simulink model "mppt1"  (R2026a)
settings: Solver=VariableStepAuto
libraries: fl_lib x9, nesl_utility x5, ee_lib x3, batt_lib x2, batteryecm_lib x1, eePwmGenerator x1
(part 1 of 2)
settings Model: Creator=Patrick  LastModifiedBy=caden

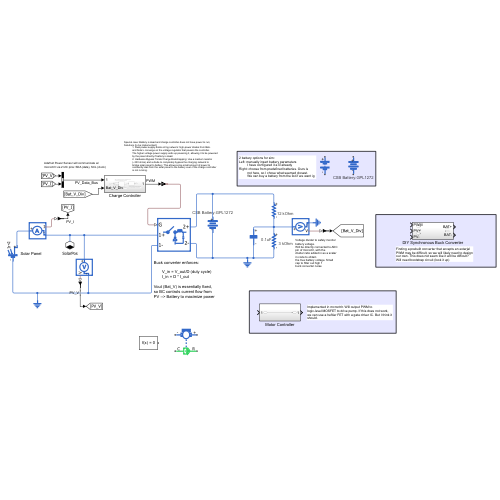
[thumbnail: Simulink's stored preview of the top-level diagram]
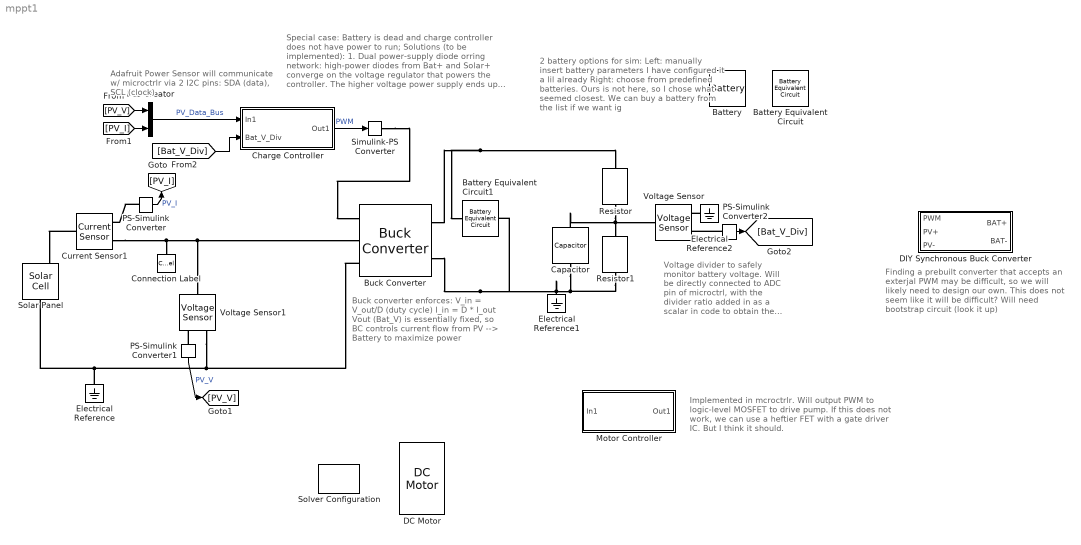
== system mppt1 ==
  note: Special case: Battery is dead and charge controller does not have power to run;
      | Solutions (to be implemented):
      | 1. Dual power-supply diode orring network: high-power diodes from Bat+
      | and Solar+ converge on the voltage regulator that powers the controller.
      | The higher voltage power supply ends up powering it, allowing it to be powered
      | by the panel directly if battery is dead.
      | 2. Hardware Bypass Trickle Charge Bootstrapping: Use a medium resistor
      | (~330 ohms) and a diode to completely bypass the charging network to
      | bridge solar panel to battery. This allows some small amount of power to
      | constantly leak from the solar panel to the battery even if the charge controller
      | is not running.
  note: Implemented in mcroctrlr. Will output PWM to
      | logic-level MOSFET to drive pump. If this does not work,
      | we can use a heftier FET with a gate driver IC. But I think it
      | should.
  note: Finding a prebuilt converter that accepts an exterjal
      | PWM may be difficult, so we will likely need to design
      | our own. This does not seem like it will be difficult?
      | Will need bootstrap circuit (look it up)
  note: Voltage divider to safely monitor battery voltage.
      | Will be directly connected to ADC pin of microctrl, with the
      | divider ratio added in as a scalar in code to obtain
      | the true battery voltage. Small cap to filter out high f
      | buck converter noise
  note: 2 battery options for sim:
      | Left: manually insert battery parameters
      | I have configured it a lil already
      | Right: choose from predefined batteries. Ours is
      | not here, so I chose what seemed closest.
      | We can buy a battery from the list if we want ig
  note: Adafruit Power Sensor will communicate w/
      | microctrlr via 2 I2C pins: SDA (data), SCL (clock)
  note: Buck converter enforces:
      |
      | 	V_in = V_out/D (duty cycle)
      | 	I_in = D * I_out
      |
      | Vout (Bat_V) is essentially fixed,
      | so BC controls current flow from
      | PV --> Battery to maximize power
  Battery : batteryecm_lib/Battery  Vnom=12 V  prm_dir=simscape.enum.battery.prm_dir.disabled  R1_dis=2 Ohm  R1_ch=2 Ohm  R1=25 mOhm  prm_AH=simscape.enum.battery.prm_AH.finite  AH=8 A*hr  V1=11 V  AH1=1.6 A*hr  prm_R2=simscape.enum.battery.prm_R2.disabled  R2=2000 Ohm  Tmeas=298.15 K  charge_measurement_port=simscape.enum.battery.enable.no  prm_dyn=simscape.enum.battery.prm_dyn.rc1  Rp1=0.005 Ohm  tau1=10 s  Rp2=0.005 Ohm  tau2=30 s  Rp3=0.005 Ohm  tau3=30 s  Rp4=0.005 Ohm  tau4=30 s  Rp5=0.005 Ohm  tau5=30 s  prm_fade=simscape.enum.battery.prm_fade.disabled  N_fade=100  AH_fade=45 A*hr  R1_fade=2.02 Ohm  R1_ch_fade=2.02 Ohm  V1_fade=10.35 V  prm_age=simscape.enum.battery.prm_age.disabled  prm_age_OCV=simscape.enum.battery.prm_age_OCV.OCV  OCV_age=0.9  SOC_age=60  Tmeas_age=298.15 K  delta_time_age_vec=[0] d  temperature_age_vec=[273] K  OCV_scaling_age=2.2134e6  OCV_offset_age=1.632e6  temp_exp_age=0.515833569 V  t_exp_age=0.75  Vnom_T2=12 V  R1_T2=2.2 Ohm  R1_T2_dis=2.2 Ohm  R1_T2_ch=2.2 Ohm  V1_T2=11.4 V  R2_T2=2200 Ohm  Rp1_T2=0.005 Ohm  tau1_T2=30 s  Rp2_T2=0.005 Ohm  tau2_T2=30 s  Rp3_T2=0.005 Ohm  tau3_T2=30 s  Rp4_T2=0.005 Ohm  tau4_T2=30 s  Rp5_T2=0.005 Ohm  tau5_T2=30 s  Tmeas2=273.15 K  thermal_port=simscape.enum.thermaleffects.omit  thermal_mass=30000 J/K  i_specify=off  i_priority=None  i=0 A  i_nominal_specify=off  i_nominal_value=1  i_nominal_unit=A  v_specify=off  v_priority=None  v=0 V  v_nominal_specify=off  v_nominal_value=1  v_nominal_unit=V  charge_specify=off  charge_priority=High  charge=50 A*hr  charge_nominal_specify=off  charge_nominal_value=1  charge_nominal_unit=A*hr  num_cycles_specify=off  num_cycles_priority=High  num_cycles=0  num_cycles_nominal_specify=off  num_cycles_nominal_value=1  num_cycles_nominal_unit=1  temperature_specify=off  temperature_priority=High  temperature=298.15 K  temperature_nominal_specify=off  temperature_nominal_value=1  temperature_nominal_unit=K
  Battery Equivalent Circuit : batt_lib/Cells/Battery Equivalent Circuit  PartSpecification="{\"CollectionId\":\"MW.SimscapeBattery\",\"CollectionVersion\":\"1.0.0\",\"DatasetId\":\"CSB Battery|GPL1272|simscape.battery.batteryEquivalentCircuit\",\"DisplayName\":\"CSB Battery:GPL1272\"}"  BatteryCapacity=7.2 % Datasheet derived hr*A  ThermalModel=simscape.battery.enum.cells.BatteryThermalModel.ConstantTemperature  ExtrapolationMethod=simscape.enum.extrapolation.linear  SOCBreakpoints=[0 0.02 0.04 0.06 0.08 0.1 0.12 0.14 0.16 0.18 0.2 0.22 0.24 0.26 0.28 0.3 0.32 0.34 0.36 0.38 0.4 0.42 0.44 0.46 0.48 0.5 0.52 0.54 0.56 0.58 0.6 0.62 0.64 0.66 0.68 0.7 0.72 0.74 0.76 0.78 0.8 0.82 0.84 0.86 0.88 0.9 0.92 0.94 0.96 0.98 1] % Datasheet derived  TemperatureBreakpoints=[25;30] % Parameter assumed degC  OpenCircuitVoltage=[10.55448 10.75925 10.91906 11.06757 11.18985 11.28642 11.36577 11.43656 11.50322 11.56016 11.61342 11.66505 11.71348 11.75917 11.80784 11.85717 11.90449 11.94971 11.9929 12.03397 12.07275 12.10969 12.14517 12.17949 12.21291 12.24568 12.27779 12.30916 12.3396 12.36887 12.39694 12.42373 12.4492 12.47369 12.49775 12.5218 12.54639 12.57213 12.59914 12.62744 12.65704 12.68789 12.71992 12.75327 12.78809 12.82459 12.86341 12.90404 12.94821 12.99301 13.04366] % Datasheet derived V  OpenCircuitVoltageThermal=[10.55448 10.55448;10.75925 10.75925;10.91906 10.91906;11.06757 11.06757;11.18985 11.18985;11.28642 11.28642;11.36577 11.36577;11.43656 11.43656;11.50322 11.50322;11.56016 11.56016;11.61342 11.61342;11.66505 11.66505;11.71348 11.71348;11.75917 11.75917;11.80784 11.80784;11.85717 11.85717;11.90449 11.90449;11.94971 11.94971;11.9929 11.9929;12.03397 12.03397;12.07275 12.07275;12.10969 12.10969;12.14517 12.14517;12.17949 12.17949;12.21291 12.21291;12.24568 12.24568;12.27779 12.27779;12.30916 12.30916;12.3396 12.3396;12.36887 12.36887;12.39694 12.39694;12.42373 12.42373;12.4492 12.4492;12.47369 12.47369;12.49775 12.49775;12.5218 12.5218;12.54639 12.54639;12.57213 12.57213;12.59914 12.59914;12.62744 12.62744;12.65704 12.65704;12.68789 12.68789;12.71992 12.71992;12.75327 12.75327;12.78809 12.78809;12.82459 12.82459;12.86341 12.86341;12.90404 12.90404;12.94821 12.94821;12.99301 12.99301;13.04366 13.04366] % Parameter assumed V  VoltageRange=[9.45 Inf] % Datasheet derived V  HysteresisModel=simscape.battery.enum.cells.HysteresisModel.none  MaximumHysteresisVoltage=[0, 0, 0, 0, 0, 0, 0] % Parameter not set V  InstantaneousHysteresisVoltage=[0, 0, 0, 0, 0, 0, 0] % Parameter not set V  HysteresisRate=0.1 % Parameter not set  MaximumHysteresisVoltageThermal=[0, 0, 0; 0, 0, 0; 0, 0, 0; 0, 0, 0; 0, 0, 0; 0, 0, 0; 0, 0, 0] % Parameter not set V  InstantaneousHysteresisVoltageThermal=[0, 0, 0; 0, 0, 0; 0, 0, 0; 0, 0, 0; 0, 0, 0; 0, 0, 0; 0, 0, 0] % Parameter not set V  HysteresisRateThermal=0.1 % Parameter not set  ResistanceSOCBreakpoints=[0 0.02 0.04 0.06 0.08 0.1 0.12 0.14 0.16 0.18 0.2 0.22 0.24 0.26 0.28 0.3 0.32 0.34 0.36 0.38 0.4 0.42 0.44 0.46 0.48 0.5 0.52 0.54 0.56 0.58 0.6 0.62 0.64 0.66 0.68 0.7 0.72 0.74 0.76 0.78 0.8 0.82 0.84 0.86 0.88 0.9 0.92 0.94 0.96 0.98 1] % Datasheet derived  ResistanceTemperatureBreakpoints=[25;30] % Parameter assumed degC  ResistanceCurrentBreakpoints=[-1, 0, 1] % Parameter not set A  CurrentDependence=simscape.battery.enum.cells.CurrentDependence.Disabled  R0=[0.4783 0.48483 0.48048 0.47338 0.45841 0.43749 0.41141 0.38282 0.35427 0.32759 0.3043 0.2847 0.26811 0.25342 0.23949 0.22498 0.20981 0.19439 0.17947 0.16593 0.15482 0.14608 0.13938 0.13434 0.13049 0.12727 0.12445 0.12176 0.11887 0.11543 0.11119 0.10615 0.1005 0.09461 0.08893 0.08388 0.07966 0.0763 0.07371 0.07171 0.07009 0.0687 0.06744 0.06622 0.06513 0.06423 0.06395 0.06429 0.06617 0.06825 0.07319] % Datasheet derived Ohm  R0I=[.0117, .0085, .009; .011, .0085, .009; .0114, .0087, .0092; .0107, .0082, .0088; .0107, .0083, .0091; .0113, .0085, .0089; .0116, .0085, .0089] % Parameter not set Ohm  R0Thermal=[0.4783 0.4783;0.48483 0.48483;0.48048 0.48048;0.47338 0.47338;0.45841 0.45841;0.43749 0.43749;0.41141 0.41141;0.38282 0.38282;0.35427 0.35427;0.32759 0.32759;0.3043 0.3043;0.2847 0.2847;0.26811 0.26811;0.25342 0.25342;0.23949 0.23949;0.22498 0.22498;0.20981 0.20981;0.19439 0.19439;0.17947 0.17947;0.16593 0.16593;0.15482 0.15482;0.14608 0.14608;0.13938 0.13938;0.13434 0.13434;0.13049 0.13049;0.12727 0.12727;0.12445 0.12445;0.12176 0.12176;0.11887 0.11887;0.11543 0.11543;0.11119 0.11119;0.10615 0.10615;0.1005 0.1005;0.09461 0.09461;0.08893 0.08893;0.08388 0.08388;0.07966 0.07966;0.0763 0.0763;0.07371 0.07371;0.07171 0.07171;0.07009 0.07009;0.0687 0.0687;0.06744 0.06744;0.06622 0.06622;0.06513 0.06513;0.06423 0.06423;0.06395 0.06395;0.06429 0.06429;0.06617 0.06617;0.06825 0.06825;0.07319 0.07319] % Parameter assumed Ohm  R0ThermalI=repmat([.0117, .0085, .009; .011, .0085, .009; .0114, .0087, .0092; .0107, .0082, .0088; .0107, .0083, .0091; .0113, .0085, .0089; .0116, .0085, .0089], 1, 1, 3) % Parameter not set Ohm  DischargeR0=[.0085, .0085, .0087, .0082, .0083, .0085, .0085] % Parameter not set Ohm  ChargeR0=[.0085, .0085, .0087, .0082, .0083, .0085, .0085] % Parameter not set Ohm  ChargeR0Thermal=[.0117, .0085, .009; .011, .0085, .009; .0114, .0087, .0092; .0107, .0082, .0088; .0107, .0083, .0091; .0113, .0085, .0089; .0116, .0085, .0089] % Parameter not set Ohm  DischargeR0Thermal=[.0117, .0085, .009; .011, .0085, .009; .0114, .0087, .0092; .0107, .0082, .0088; .0107, .0083, .0091; .0113, .0085, .0089; .0116, .0085, .0089] % Parameter not set Ohm  RCPairs=simscape.battery.enum.cells.RCPairs.noDynamics  R1=[.0029, .0024, .0026, .0016, .0023, .0018, .0017] % Parameter not set Ohm  Tau1=[36, 45, 105, 29, 77, 33, 39] % Parameter not set s  R2=[.0029, .0024, .0026, .0016, .0023, .0018, .0017] % Parameter not set Ohm  Tau2=[36, 45, 105, 29, 77, 33, 39] % Parameter not set s  R3=[.0029, .0024, .0026, .0016, .0023, .0018, .0017] % Parameter not set Ohm  Tau3=[36, 45, 105, 29, 77, 33, 39] % Parameter not set s  R1I=[.0109, .0029, .0013; .0069, .0024, .0012; .0047, .0026, .0013; .0034, .0016, .001; .0033, .0023, .0014; .0033, .0018, .0011; .0028, .0017, .0011] % Parameter not set Ohm  Tau1I=[20, 36, 39; 31, 45, 39; 109, 105, 61; 36, 29, 26; 59, 77, 67; 40, 33, 29; 25, 39, 33] % Parameter not set s  R2I=[.0109, .0029, .0013; .0069, .0024, .0012; .0047, .0026, .0013; .0034, .0016, .001; .0033, .0023, .0014; .0033, .0018, .0011; .0028, .0017, .0011] % Parameter not set Ohm  Tau2I=[20, 36, 39; 31, 45, 39; 109, 105, 61; 36, 29, 26; 59, 77, 67; 40, 33, 29; 25, 39, 33] % Parameter not set s  R3I=[.0109, .0029, .0013; .0069, .0024, .0012; .0047, .0026, .0013; .0034, .0016, .001; .0033, .0023, .0014; .0033, .0018, .0011; .0028, .0017, .0011] % Parameter not set Ohm  Tau3I=[20, 36, 39; 31, 45, 39; 109, 105, 61; 36, 29, 26; 59, 77, 67; 40, 33, 29; 25, 39, 33] % Parameter not set s  DischargeR1=[.0029, .0024, .0026, .0016, .0023, .0018, .0017] % Parameter not set Ohm  DischargeTau1=[36, 45, 105, 29, 77, 33, 39] % Parameter not set s  ChargeR1=[.0029, .0024, .0026, .0016, .0023, .0018, .0017] % Parameter not set Ohm  ChargeTau1=[36, 45, 105, 29, 77, 33, 39] % Parameter not set s  DischargeR2=[.0029, .0024, .0026, .0016, .0023, .0018, .0017] % Parameter not set Ohm  DischargeTau2=[36, 45, 105, 29, 77, 33, 39] % Parameter not set s  ChargeR2=[.0029, .0024, .0026, .0016, .0023, .0018, .0017] % Parameter not set Ohm  ChargeTau2=[36, 45, 105, 29, 77, 33, 39] % Parameter not set s  DischargeR3=[.0029, .0024, .0026, .0016, .0023, .0018, .0017] % Parameter not set Ohm  DischargeTau3=[36, 45, 105, 29, 77, 33, 39] % Parameter not set s  ChargeR3=[.0029, .0024, .0026, .0016, .0023, .0018, .0017] % Parameter not set Ohm  ChargeTau3=[36, 45, 105, 29, 77, 33, 39] % Parameter not set s  R1Thermal=[.0109, .0029, .0013; .0069, .0024, .0012; .0047, .0026, .0013; .0034, .0016, .001; .0033, .0023, .0014; .0033, .0018, .0011; .0028, .0017, .0011] % Parameter not set Ohm  Tau1Thermal=[20, 36, 39; 31, 45, 39; 109, 105, 61; 36, 29, 26; 59, 77, 67; 40, 33, 29; 25, 39, 33] % Parameter not set s  R2Thermal=[.0109, .0029, .0013; .0069, .0024, .0012; .0047, .0026, .0013; .0034, .0016, .001; .0033, .0023, .0014; .0033, .0018, .0011; .0028, .0017, .0011] % Parameter not set Ohm  Tau2Thermal=[20, 36, 39; 31, 45, 39; 109, 105, 61; 36, 29, 26; 59, 77, 67; 40, 33, 29; 25, 39, 33] % Parameter not set s  R3Thermal=[.0109, .0029, .0013; .0069, .0024, .0012; .0047, .0026, .0013; .0034, .0016, .001; .0033, .0023, .0014; .0033, .0018, .0011; .0028, .0017, .0011] % Parameter not set Ohm  Tau3Thermal=[20, 36, 39; 31, 45, 39; 109, 105, 61; 36, 29, 26; 59, 77, 67; 40, 33, 29; 25, 39, 33] % Parameter not set s  R1ThermalI=repmat([.0109, .0029, .0013; .0069, .0024, .0012; .0047, .0026, .0013; .0034, .0016, .001; .0033, .0023, .0014; .0033, .0018, .0011; .0028, .0017, .0011], 1, 1, 3) % Parameter not set Ohm  Tau1ThermalI=repmat([20, 36, 39; 31, 45, 39; 109, 105, 61; 36, 29, 26; 59, 77, 67; 40, 33, 29; 25, 39, 33], 1, 1, 3) % Parameter not set s  R2ThermalI=repmat([.0109, .0029, .0013; .0069, .0024, .0012; .0047, .0026, .0013; .0034, .0016, .001; .0033, .0023, .0014; .0033, .0018, .0011; .0028, .0017, .0011], 1, 1, 3) % Parameter not set Ohm  Tau2ThermalI=repmat([20, 36, 39; 31, 45, 39; 109, 105, 61; 36, 29, 26; 59, 77, 67; 40, 33, 29; 25, 39, 33], 1, 1, 3) % Parameter not set s  R3ThermalI=repmat([.0109, .0029, .0013; .0069, .0024, .0012; .0047, .0026, .0013; .0034, .0016, .001; .0033, .0023, .0014; .0033, .0018, .0011; .0028, .0017, .0011], 1, 1, 3) % Parameter not set Ohm  Tau3ThermalI=repmat([20, 36, 39; 31, 45, 39; 109, 105, 61; 36, 29, 26; 59, 77, 67; 40, 33, 29; 25, 39, 33], 1, 1, 3) % Parameter not set s  DischargeR1Thermal=[.0109, .0029, .0013; .0069, .0024, .0012; .0047, .0026, .0013; .0034, .0016, .001; .0033, .0023, .0014; .0033, .0018, .0011; .0028, .0017, .0011] % Parameter not set Ohm  DischargeTau1Thermal=[20, 36, 39; 31, 45, 39; 109, 105, 61; 36, 29, 26; 59, 77, 67; 40, 33, 29; 25, 39, 33] % Parameter not set s  ChargeR1Thermal=[.0109, .0029, .0013; .0069, .0024, .0012; .0047, .0026, .0013; .0034, .0016, .001; .0033, .0023, .0014; .0033, .0018, .0011; .0028, .0017, .0011] % Parameter not set Ohm  ChargeTau1Thermal=[20, 36, 39; 31, 45, 39; 109, 105, 61; 36, 29, 26; 59, 77, 67; 40, 33, 29; 25, 39, 33] % Parameter not set s  DischargeR2Thermal=[.0109, .0029, .0013; .0069, .0024, .0012; .0047, .0026, .0013; .0034, .0016, .001; .0033, .0023, .0014; .0033, .0018, .0011; .0028, .0017, .0011] % Parameter not set Ohm  DischargeTau2Thermal=[20, 36, 39; 31, 45, 39; 109, 105, 61; 36, 29, 26; 59, 77, 67; 40, 33, 29; 25, 39, 33] % Parameter not set s  ChargeR2Thermal=[.0109, .0029, .0013; .0069, .0024, .0012; .0047, .0026, .0013; .0034, .0016, .001; .0033, .0023, .0014; .0033, .0018, .0011; .0028, .0017, .0011] % Parameter not set Ohm  ChargeTau2Thermal=[20, 36, 39; 31, 45, 39; 109, 105, 61; 36, 29, 26; 59, 77, 67; 40, 33, 29; 25, 39, 33] % Parameter not set s  DischargeR3Thermal=[.0109, .0029, .0013; .0069, .0024, .0012; .0047, .0026, .0013; .0034, .0016, .001; .0033, .0023, .0014; .0033, .0018, .0011; .0028, .0017, .0011] % Parameter not set Ohm  DischargeTau3Thermal=[20, 36, 39; 31, 45, 39; 109, 105, 61; 36, 29, 26; 59, 77, 67; 40, 33, 29; 25, 39, 33] % Parameter not set s  ChargeR3Thermal=[.0109, .0029, .0013; .0069, .0024, .0012; .0047, .0026, .0013; .0034, .0016, .001; .0033, .0023, .0014; .0033, .0018, .0011; .0028, .0017, .0011] % Parameter not set Ohm  ChargeTau3Thermal=[20, 36, 39; 31, 45, 39; 109, 105, 61; 36, 29, 26; 59, 77, 67; 40, 33, 29; 25, 39, 33] % Parameter not set s  SelfDischargeResistor=simscape.battery.enum.cells.BatteryEnable.Disabled  SelfDischargeR=7e3 % Parameter not set Ohm  SelfDischargeRThermal=[8000, 7000, 6000] % Parameter not set Ohm  CyclingAgingMethod=simscape.battery.enum.cells.CyclingAgingMethod.tableN  CycleCalculationMethod=simscape.battery.enum.cells.CycleCalculationMethod.EquivalentCycles  NumDisCycles=100 % Parameter not set  OCVChange=0 % Parameter not set  R0Change=0 % Parameter not set  CapacityChange=0 % Parameter not set  SelfDischargeRChange=0 % Parameter not set  R1Change=0 % Parameter not set  R2Change=0 % Parameter not set  R3Change=0 % Parameter not set  NumDisCyclesBreakpoints=[1 63 125 187 249 311 373 435 497 559 621 683 745 807 869 931 993 1055 1117 1179] % Datasheet derived  AgingTemperatureBreakpoints=[298.15, 323.15] % Parameter not set K  AgingCurrentBreakpoints=[-.1, -.5, -5] % Parameter not set A  OCVChangeVec=[0.0315 0.5992 0.9059 1.0322 1.0661 0.9389 0.7283 0.4511 0.0588 -0.3759 -0.8078 -1.2378 -1.6654 -2.0898 -2.5151 -2.9295 -3.3394 -3.738 -4.1399 -4.584] % Parameter assumed  OCVChangeThermal=[0, 0; 0, 0; 0, 0; 0, 0] % Parameter not set  R0ChangeVec=[0 0 0 0 0 0 0 0 0 0 0 0 0 0 0 0 0 0 0 0] % Parameter assumed  R0ChangeThermal=[0, 0; 0, 0; 0, 0; 0, 0] % Parameter not set  R0ChangeThermalI=repmat(0, 4, 2, 3) % Parameter not set  R0CyclingChangeInitialTarget=0 % Parameter not set  CapacityChangeVec=[-5.051 -2.279 -0.782 -0.165 0 -0.621 -1.649 -3.003 -4.918 -7.041 -9.423 -11.912 -14.595 -17.507 -20.628 -23.887 -27.357 -31.033 -35.073 -39.589] % Datasheet derived  CapacityChangeThermal=[0, 0; 0, 0; 0, 0; 0, 0] % Parameter not set  CapacityChangeThermalI=repmat(0, 4, 2, 3) % Parameter not set  CapacityCyclingChangeInitialTarget=0 % Parameter not set  SelfDischargeRChangeVec=[0, 0, 0, 0] % Parameter not set  SelfDischargeRChangeThermal=[0, 0; 0, 0; 0, 0; 0, 0] % Parameter not set  SelfDischargeRChangeThermalI=repmat(0, 4, 2, 3) % Parameter not set  SelfDischargeRCyclingChangeInitialTarget=0 % Parameter not set  R1ChangeVec=[0, 0, 0, 0] % Parameter not set  R1ChangeThermal=[0, 0; 0, 0; 0, 0; 0, 0] % Parameter not set  R1ChangeThermalI=repmat(0, 4, 2, 3) % Parameter not set  R1CyclingChangeInitialTarget=0 % Parameter not set  R2ChangeVec=[0, 0, 0, 0] % Parameter not set  R2ChangeThermal=[0, 0; 0, 0; 0, 0; 0, 0] % Parameter not set  R2ChangeThermalI=repmat(0, 4, 2, 3) % Parameter not set  R2CyclingChangeInitialTarget=0 % Parameter not set  R3ChangeVec=[0, 0, 0, 0] % Parameter not set  R3ChangeThermal=[0, 0; 0, 0; 0, 0; 0, 0] % Parameter not set  R3ChangeThermalI=repmat(0, 4, 2, 3) % Parameter not set  R3CyclingChangeInitialTarget=0 % Parameter not set  CalendarAgeResistance=simscape.battery.enum.cells.BatteryEnable.Disabled  CalendarAgeCapacity=simscape.battery.enum.cells.BatteryEnable.Enabled  CalendarAgingMethod=simscape.battery.enum.cells.CalendarAgingMethod.tableTandTime  StorageVariable=simscape.battery.enum.cells.StorageVariable.OCV  OCVDuringStorage=0.9 % Parameter not set  SOCDuringStorage=0.6 % Parameter not set  StorageTimeIntervals=0 % Parameter not set d  StorageTemperatures=273 % Parameter not set K  ResistanceScalingOCV=2.2134e6 % Parameter not set  ResistanceScalingOCVOffset=1.632e6 % Parameter not set  ResistanceExponentialIncrease=0.515833569 % Parameter not set V  ResistanceTimeExponent=0.75 % Parameter not set  ResistanceAgeTemperatureBreakpoints=[273.15, 298.15, 323.15] % Parameter not set K  ResistanceAgeTimeBreakpoints=[0, 90, 180, 270] % Parameter not set d  PercentResistanceChange=[0, 0, 0] % Parameter not set  ResistanceTimeBreakpoints=100 % Parameter not set d  PercentResistanceChangeThermal=[0, 0, 0; 0, 0, 0; 0, 0, 0; 0, 0, 0] % Parameter not set  CapacityScalingOCV=1.5097e07 % Parameter not set  CapacityScalingOCVOffset=8.3625e06 % Parameter not set  CapacityExponentialIncrease=0.6011 % Parameter not set V  CapacityTimeExponent=0.75 % Parameter not set  CapacityAgeTemperatureBreakpoints=[5 25 30 40] % Datasheet derived degC  CapacityAgeTimeBreakpoints=[1 29 57 85 113 141 169 197 225 253 281 309 337 365 393 421 449 477 505 533 561] % Datasheet derived d  PercentCapacityChange=[0, 0, 0] % Parameter not set  CapacityTimeBreakpoints=100 % Parameter not set d  PercentCapacityChangeThermal=[-12.16003 -12.05239 -12.1695 -12.09683;-12.86337 -14.52728 -16.99685 -20.72464;-13.70598 -17.13684 -21.40096 -27.85651;-14.55234 -19.69649 -25.62782 -33.8946;-15.39921 -22.17854 -29.53628 -39.21373;-16.25192 -24.59585 -33.26735 -43.824;-17.06738 -27.04531 -36.69448 -48.04282;-17.84583 -29.39901 -39.91743 -51.10766;-18.67228 -31.83985 -42.90723 -53.76751;-19.4824 -34.22411 -45.64728 -56.42735;-20.29628 -36.48052 -48.11969 -59.0872;-21.15972 -38.79001 -50.6323 -61.74704;-21.98269 -40.98584 -53.11668 -64.40688;-22.7952 -43.14859 -55.60106 -67.06673;-23.58639 -45.35431 -58.08544 -69.72657;-24.41788 -47.50229 -60.56983 -72.38642;-25.26019 -49.69778 -63.05421 -75.04626;-26.10099 -51.98571 -65.53859 -77.7061;-26.91077 -54.29114 -68.02297 -80.36595;-27.73583 -56.59657 -70.50735 -83.02579;-28.55906 -58.902 -72.99173 -85.68564]  SimulationTemperature=298.15 % Parameter not set K  BatteryThermalMass=2340 % Parameter assumed J/K  NumThermalModels=6 % Parameter not set  ThermalConductivityZ=18 % Parameter not set W/(K*m)  CrossSectionalAreaXY=9784.8 % Datasheet derived mm^2  Height=94.3 % Datasheet derived mm  ReversibleHeatModel=simscape.battery.enum.cells.ReversibleHeatModel.Disabled  EntropicCoefficient=[0, 0, 0, 0, 0, 0, 0] % Parameter not set mV/K  CurrentDirectionality=simscape.battery.enum.cells.BatteryEnable.Disabled  stateOfCharge_specify=off  stateOfCharge_priority=High  stateOfCharge=1  stateOfCharge_nominal_specify=off  stateOfCharge_nominal_value=1  stateOfCharge_nominal_unit=1  batteryVoltage_specify=off  batteryVoltage_priority=None  batteryVoltage=0 V  batteryVoltage_nominal_specify=off  batteryVoltage_nominal_value=1  batteryVoltage_nominal_unit=V  batteryCurrent_specify=off  batteryCurrent_priority=None  batteryCurrent=0 A  batteryCurrent_nominal_specify=off  batteryCurrent_nominal_value=1  batteryCurrent_nominal_unit=A  numCycles_specify=off  numCycles_priority=High  numCycles=0  numCycles_nominal_specify=off  numCycles_nominal_value=1  numCycles_nominal_unit=1  batteryTemperature_specify=off  batteryTemperature_priority=High  batteryTemperature=298.15 K  batteryTemperature_nominal_specify=off  batteryTemperature_nominal_value=1  batteryTemperature_nominal_unit=K  hysteresisState_specify=off  hysteresisState_priority=High  hysteresisState=0  hysteresisState_nominal_specify=off  hysteresisState_nominal_value=1  hysteresisState_nominal_unit=1  isExothermFaulted_specify=off  isExothermFaulted_priority=None  isExothermFaulted=0  isExothermFaulted_nominal_specify=off  isExothermFaulted_nominal_value=1  isExothermFaulted_nominal_unit=1  reactionHeatRate_specify=off  reactionHeatRate_priority=None  reactionHeatRate=0 W  reactionHeatRate_nominal_specify=off  reactionHeatRate_nominal_value=1  reactionHeatRate_nominal_unit=W  reactionExtent_specify=off  reactionExtent_priority=None  reactionExtent=0  reactionExtent_nominal_specify=off  reactionExtent_nominal_value=1  reactionExtent_nominal_unit=1
      settings: AttributesFormatString=CSB Battery:GPL1272
  Battery Equivalent Circuit1 : batt_lib/Cells/Battery Equivalent Circuit  PartSpecification="{\"CollectionId\":\"MW.SimscapeBattery\",\"CollectionVersion\":\"1.0.0\",\"DatasetId\":\"CSB Battery|GPL1272|simscape.battery.batteryEquivalentCircuit\",\"DisplayName\":\"CSB Battery:GPL1272\"}"  BatteryCapacity=7.2 % Datasheet derived hr*A  ThermalModel=simscape.battery.enum.cells.BatteryThermalModel.ConstantTemperature  ExtrapolationMethod=simscape.enum.extrapolation.linear  SOCBreakpoints=[0 0.02 0.04 0.06 0.08 0.1 0.12 0.14 0.16 0.18 0.2 0.22 0.24 0.26 0.28 0.3 0.32 0.34 0.36 0.38 0.4 0.42 0.44 0.46 0.48 0.5 0.52 0.54 0.56 0.58 0.6 0.62 0.64 0.66 0.68 0.7 0.72 0.74 0.76 0.78 0.8 0.82 0.84 0.86 0.88 0.9 0.92 0.94 0.96 0.98 1] % Datasheet derived  TemperatureBreakpoints=[25;30] % Parameter assumed degC  OpenCircuitVoltage=[10.55448 10.75925 10.91906 11.06757 11.18985 11.28642 11.36577 11.43656 11.50322 11.56016 11.61342 11.66505 11.71348 11.75917 11.80784 11.85717 11.90449 11.94971 11.9929 12.03397 12.07275 12.10969 12.14517 12.17949 12.21291 12.24568 12.27779 12.30916 12.3396 12.36887 12.39694 12.42373 12.4492 12.47369 12.49775 12.5218 12.54639 12.57213 12.59914 12.62744 12.65704 12.68789 12.71992 12.75327 12.78809 12.82459 12.86341 12.90404 12.94821 12.99301 13.04366] % Datasheet derived V  OpenCircuitVoltageThermal=[10.55448 10.55448;10.75925 10.75925;10.91906 10.91906;11.06757 11.06757;11.18985 11.18985;11.28642 11.28642;11.36577 11.36577;11.43656 11.43656;11.50322 11.50322;11.56016 11.56016;11.61342 11.61342;11.66505 11.66505;11.71348 11.71348;11.75917 11.75917;11.80784 11.80784;11.85717 11.85717;11.90449 11.90449;11.94971 11.94971;11.9929 11.9929;12.03397 12.03397;12.07275 12.07275;12.10969 12.10969;12.14517 12.14517;12.17949 12.17949;12.21291 12.21291;12.24568 12.24568;12.27779 12.27779;12.30916 12.30916;12.3396 12.3396;12.36887 12.36887;12.39694 12.39694;12.42373 12.42373;12.4492 12.4492;12.47369 12.47369;12.49775 12.49775;12.5218 12.5218;12.54639 12.54639;12.57213 12.57213;12.59914 12.59914;12.62744 12.62744;12.65704 12.65704;12.68789 12.68789;12.71992 12.71992;12.75327 12.75327;12.78809 12.78809;12.82459 12.82459;12.86341 12.86341;12.90404 12.90404;12.94821 12.94821;12.99301 12.99301;13.04366 13.04366] % Parameter assumed V  VoltageRange=[9.45 Inf] % Datasheet derived V  HysteresisModel=simscape.battery.enum.cells.HysteresisModel.none  MaximumHysteresisVoltage=[0, 0, 0, 0, 0, 0, 0] % Parameter not set V  InstantaneousHysteresisVoltage=[0, 0, 0, 0, 0, 0, 0] % Parameter not set V  HysteresisRate=0.1 % Parameter not set  MaximumHysteresisVoltageThermal=[0, 0, 0; 0, 0, 0; 0, 0, 0; 0, 0, 0; 0, 0, 0; 0, 0, 0; 0, 0, 0] % Parameter not set V  InstantaneousHysteresisVoltageThermal=[0, 0, 0; 0, 0, 0; 0, 0, 0; 0, 0, 0; 0, 0, 0; 0, 0, 0; 0, 0, 0] % Parameter not set V  HysteresisRateThermal=0.1 % Parameter not set  ResistanceSOCBreakpoints=[0 0.02 0.04 0.06 0.08 0.1 0.12 0.14 0.16 0.18 0.2 0.22 0.24 0.26 0.28 0.3 0.32 0.34 0.36 0.38 0.4 0.42 0.44 0.46 0.48 0.5 0.52 0.54 0.56 0.58 0.6 0.62 0.64 0.66 0.68 0.7 0.72 0.74 0.76 0.78 0.8 0.82 0.84 0.86 0.88 0.9 0.92 0.94 0.96 0.98 1] % Datasheet derived  ResistanceTemperatureBreakpoints=[25;30] % Parameter assumed degC  ResistanceCurrentBreakpoints=[-1, 0, 1] % Parameter not set A  CurrentDependence=simscape.battery.enum.cells.CurrentDependence.Disabled  R0=[0.4783 0.48483 0.48048 0.47338 0.45841 0.43749 0.41141 0.38282 0.35427 0.32759 0.3043 0.2847 0.26811 0.25342 0.23949 0.22498 0.20981 0.19439 0.17947 0.16593 0.15482 0.14608 0.13938 0.13434 0.13049 0.12727 0.12445 0.12176 0.11887 0.11543 0.11119 0.10615 0.1005 0.09461 0.08893 0.08388 0.07966 0.0763 0.07371 0.07171 0.07009 0.0687 0.06744 0.06622 0.06513 0.06423 0.06395 0.06429 0.06617 0.06825 0.07319] % Datasheet derived Ohm  R0I=[.0117, .0085, .009; .011, .0085, .009; .0114, .0087, .0092; .0107, .0082, .0088; .0107, .0083, .0091; .0113, .0085, .0089; .0116, .0085, .0089] % Parameter not set Ohm  R0Thermal=[0.4783 0.4783;0.48483 0.48483;0.48048 0.48048;0.47338 0.47338;0.45841 0.45841;0.43749 0.43749;0.41141 0.41141;0.38282 0.38282;0.35427 0.35427;0.32759 0.32759;0.3043 0.3043;0.2847 0.2847;0.26811 0.26811;0.25342 0.25342;0.23949 0.23949;0.22498 0.22498;0.20981 0.20981;0.19439 0.19439;0.17947 0.17947;0.16593 0.16593;0.15482 0.15482;0.14608 0.14608;0.13938 0.13938;0.13434 0.13434;0.13049 0.13049;0.12727 0.12727;0.12445 0.12445;0.12176 0.12176;0.11887 0.11887;0.11543 0.11543;0.11119 0.11119;0.10615 0.10615;0.1005 0.1005;0.09461 0.09461;0.08893 0.08893;0.08388 0.08388;0.07966 0.07966;0.0763 0.0763;0.07371 0.07371;0.07171 0.07171;0.07009 0.07009;0.0687 0.0687;0.06744 0.06744;0.06622 0.06622;0.06513 0.06513;0.06423 0.06423;0.06395 0.06395;0.06429 0.06429;0.06617 0.06617;0.06825 0.06825;0.07319 0.07319] % Parameter assumed Ohm  R0ThermalI=repmat([.0117, .0085, .009; .011, .0085, .009; .0114, .0087, .0092; .0107, .0082, .0088; .0107, .0083, .0091; .0113, .0085, .0089; .0116, .0085, .0089], 1, 1, 3) % Parameter not set Ohm  DischargeR0=[.0085, .0085, .0087, .0082, .0083, .0085, .0085] % Parameter not set Ohm  ChargeR0=[.0085, .0085, .0087, .0082, .0083, .0085, .0085] % Parameter not set Ohm  ChargeR0Thermal=[.0117, .0085, .009; .011, .0085, .009; .0114, .0087, .0092; .0107, .0082, .0088; .0107, .0083, .0091; .0113, .0085, .0089; .0116, .0085, .0089] % Parameter not set Ohm  DischargeR0Thermal=[.0117, .0085, .009; .011, .0085, .009; .0114, .0087, .0092; .0107, .0082, .0088; .0107, .0083, .0091; .0113, .0085, .0089; .0116, .0085, .0089] % Parameter not set Ohm  RCPairs=simscape.battery.enum.cells.RCPairs.noDynamics  R1=[.0029, .0024, .0026, .0016, .0023, .0018, .0017] % Parameter not set Ohm  Tau1=[36, 45, 105, 29, 77, 33, 39] % Parameter not set s  R2=[.0029, .0024, .0026, .0016, .0023, .0018, .0017] % Parameter not set Ohm  Tau2=[36, 45, 105, 29, 77, 33, 39] % Parameter not set s  R3=[.0029, .0024, .0026, .0016, .0023, .0018, .0017] % Parameter not set Ohm  Tau3=[36, 45, 105, 29, 77, 33, 39] % Parameter not set s  R1I=[.0109, .0029, .0013; .0069, .0024, .0012; .0047, .0026, .0013; .0034, .0016, .001; .0033, .0023, .0014; .0033, .0018, .0011; .0028, .0017, .0011] % Parameter not set Ohm  Tau1I=[20, 36, 39; 31, 45, 39; 109, 105, 61; 36, 29, 26; 59, 77, 67; 40, 33, 29; 25, 39, 33] % Parameter not set s  R2I=[.0109, .0029, .0013; .0069, .0024, .0012; .0047, .0026, .0013; .0034, .0016, .001; .0033, .0023, .0014; .0033, .0018, .0011; .0028, .0017, .0011] % Parameter not set Ohm  Tau2I=[20, 36, 39; 31, 45, 39; 109, 105, 61; 36, 29, 26; 59, 77, 67; 40, 33, 29; 25, 39, 33] % Parameter not set s  R3I=[.0109, .0029, .0013; .0069, .0024, .0012; .0047, .0026, .0013; .0034, .0016, .001; .0033, .0023, .0014; .0033, .0018, .0011; .0028, .0017, .0011] % Parameter not set Ohm  Tau3I=[20, 36, 39; 31, 45, 39; 109, 105, 61; 36, 29, 26; 59, 77, 67; 40, 33, 29; 25, 39, 33] % Parameter not set s  DischargeR1=[.0029, .0024, .0026, .0016, .0023, .0018, .0017] % Parameter not set Ohm  DischargeTau1=[36, 45, 105, 29, 77, 33, 39] % Parameter not set s  ChargeR1=[.0029, .0024, .0026, .0016, .0023, .0018, .0017] % Parameter not set Ohm  ChargeTau1=[36, 45, 105, 29, 77, 33, 39] % Parameter not set s  DischargeR2=[.0029, .0024, .0026, .0016, .0023, .0018, .0017] % Parameter not set Ohm  DischargeTau2=[36, 45, 105, 29, 77, 33, 39] % Parameter not set s  ChargeR2=[.0029, .0024, .0026, .0016, .0023, .0018, .0017] % Parameter not set Ohm  ChargeTau2=[36, 45, 105, 29, 77, 33, 39] % Parameter not set s  DischargeR3=[.0029, .0024, .0026, .0016, .0023, .0018, .0017] % Parameter not set Ohm  DischargeTau3=[36, 45, 105, 29, 77, 33, 39] % Parameter not set s  ChargeR3=[.0029, .0024, .0026, .0016, .0023, .0018, .0017] % Parameter not set Ohm  ChargeTau3=[36, 45, 105, 29, 77, 33, 39] % Parameter not set s  R1Thermal=[.0109, .0029, .0013; .0069, .0024, .0012; .0047, .0026, .0013; .0034, .0016, .001; .0033, .0023, .0014; .0033, .0018, .0011; .0028, .0017, .0011] % Parameter not set Ohm  Tau1Thermal=[20, 36, 39; 31, 45, 39; 109, 105, 61; 36, 29, 26; 59, 77, 67; 40, 33, 29; 25, 39, 33] % Parameter not set s  R2Thermal=[.0109, .0029, .0013; .0069, .0024, .0012; .0047, .0026, .0013; .0034, .0016, .001; .0033, .0023, .0014; .0033, .0018, .0011; .0028, .0017, .0011] % Parameter not set Ohm  Tau2Thermal=[20, 36, 39; 31, 45, 39; 109, 105, 61; 36, 29, 26; 59, 77, 67; 40, 33, 29; 25, 39, 33] % Parameter not set s  R3Thermal=[.0109, .0029, .0013; .0069, .0024, .0012; .0047, .0026, .0013; .0034, .0016, .001; .0033, .0023, .0014; .0033, .0018, .0011; .0028, .0017, .0011] % Parameter not set Ohm  Tau3Thermal=[20, 36, 39; 31, 45, 39; 109, 105, 61; 36, 29, 26; 59, 77, 67; 40, 33, 29; 25, 39, 33] % Parameter not set s  R1ThermalI=repmat([.0109, .0029, .0013; .0069, .0024, .0012; .0047, .0026, .0013; .0034, .0016, .001; .0033, .0023, .0014; .0033, .0018, .0011; .0028, .0017, .0011], 1, 1, 3) % Parameter not set Ohm  Tau1ThermalI=repmat([20, 36, 39; 31, 45, 39; 109, 105, 61; 36, 29, 26; 59, 77, 67; 40, 33, 29; 25, 39, 33], 1, 1, 3) % Parameter not set s  R2ThermalI=repmat([.0109, .0029, .0013; .0069, .0024, .0012; .0047, .0026, .0013; .0034, .0016, .001; .0033, .0023, .0014; .0033, .0018, .0011; .0028, .0017, .0011], 1, 1, 3) % Parameter not set Ohm  Tau2ThermalI=repmat([20, 36, 39; 31, 45, 39; 109, 105, 61; 36, 29, 26; 59, 77, 67; 40, 33, 29; 25, 39, 33], 1, 1, 3) % Parameter not set s  R3ThermalI=repmat([.0109, .0029, .0013; .0069, .0024, .0012; .0047, .0026, .0013; .0034, .0016, .001; .0033, .0023, .0014; .0033, .0018, .0011; .0028, .0017, .0011], 1, 1, 3) % Parameter not set Ohm  Tau3ThermalI=repmat([20, 36, 39; 31, 45, 39; 109, 105, 61; 36, 29, 26; 59, 77, 67; 40, 33, 29; 25, 39, 33], 1, 1, 3) % Parameter not set s  DischargeR1Thermal=[.0109, .0029, .0013; .0069, .0024, .0012; .0047, .0026, .0013; .0034, .0016, .001; .0033, .0023, .0014; .0033, .0018, .0011; .0028, .0017, .0011] % Parameter not set Ohm  DischargeTau1Thermal=[20, 36, 39; 31, 45, 39; 109, 105, 61; 36, 29, 26; 59, 77, 67; 40, 33, 29; 25, 39, 33] % Parameter not set s  ChargeR1Thermal=[.0109, .0029, .0013; .0069, .0024, .0012; .0047, .0026, .0013; .0034, .0016, .001; .0033, .0023, .0014; .0033, .0018, .0011; .0028, .0017, .0011] % Parameter not set Ohm  ChargeTau1Thermal=[20, 36, 39; 31, 45, 39; 109, 105, 61; 36, 29, 26; 59, 77, 67; 40, 33, 29; 25, 39, 33] % Parameter not set s  DischargeR2Thermal=[.0109, .0029, .0013; .0069, .0024, .0012; .0047, .0026, .0013; .0034, .0016, .001; .0033, .0023, .0014; .0033, .0018, .0011; .0028, .0017, .0011] % Parameter not set Ohm  DischargeTau2Thermal=[20, 36, 39; 31, 45, 39; 109, 105, 61; 36, 29, 26; 59, 77, 67; 40, 33, 29; 25, 39, 33] % Parameter not set s  ChargeR2Thermal=[.0109, .0029, .0013; .0069, .0024, .0012; .0047, .0026, .0013; .0034, .0016, .001; .0033, .0023, .0014; .0033, .0018, .0011; .0028, .0017, .0011] % Parameter not set Ohm  ChargeTau2Thermal=[20, 36, 39; 31, 45, 39; 109, 105, 61; 36, 29, 26; 59, 77, 67; 40, 33, 29; 25, 39, 33] % Parameter not set s  DischargeR3Thermal=[.0109, .0029, .0013; .0069, .0024, .0012; .0047, .0026, .0013; .0034, .0016, .001; .0033, .0023, .0014; .0033, .0018, .0011; .0028, .0017, .0011] % Parameter not set Ohm  DischargeTau3Thermal=[20, 36, 39; 31, 45, 39; 109, 105, 61; 36, 29, 26; 59, 77, 67; 40, 33, 29; 25, 39, 33] % Parameter not set s  ChargeR3Thermal=[.0109, .0029, .0013; .0069, .0024, .0012; .0047, .0026, .0013; .0034, .0016, .001; .0033, .0023, .0014; .0033, .0018, .0011; .0028, .0017, .0011] % Parameter not set Ohm  ChargeTau3Thermal=[20, 36, 39; 31, 45, 39; 109, 105, 61; 36, 29, 26; 59, 77, 67; 40, 33, 29; 25, 39, 33] % Parameter not set s  SelfDischargeResistor=simscape.battery.enum.cells.BatteryEnable.Disabled  SelfDischargeR=7e3 % Parameter not set Ohm  SelfDischargeRThermal=[8000, 7000, 6000] % Parameter not set Ohm  CyclingAgingMethod=simscape.battery.enum.cells.CyclingAgingMethod.tableN  CycleCalculationMethod=simscape.battery.enum.cells.CycleCalculationMethod.EquivalentCycles  NumDisCycles=100 % Parameter not set  OCVChange=0 % Parameter not set  R0Change=0 % Parameter not set  CapacityChange=0 % Parameter not set  SelfDischargeRChange=0 % Parameter not set  R1Change=0 % Parameter not set  R2Change=0 % Parameter not set  R3Change=0 % Parameter not set  NumDisCyclesBreakpoints=[1 63 125 187 249 311 373 435 497 559 621 683 745 807 869 931 993 1055 1117 1179] % Datasheet derived  AgingTemperatureBreakpoints=[298.15, 323.15] % Parameter not set K  AgingCurrentBreakpoints=[-.1, -.5, -5] % Parameter not set A  OCVChangeVec=[0.0315 0.5992 0.9059 1.0322 1.0661 0.9389 0.7283 0.4511 0.0588 -0.3759 -0.8078 -1.2378 -1.6654 -2.0898 -2.5151 -2.9295 -3.3394 -3.738 -4.1399 -4.584] % Parameter assumed  OCVChangeThermal=[0, 0; 0, 0; 0, 0; 0, 0] % Parameter not set  R0ChangeVec=[0 0 0 0 0 0 0 0 0 0 0 0 0 0 0 0 0 0 0 0] % Parameter assumed  R0ChangeThermal=[0, 0; 0, 0; 0, 0; 0, 0] % Parameter not set  R0ChangeThermalI=repmat(0, 4, 2, 3) % Parameter not set  R0CyclingChangeInitialTarget=0 % Parameter not set  CapacityChangeVec=[-5.051 -2.279 -0.782 -0.165 0 -0.621 -1.649 -3.003 -4.918 -7.041 -9.423 -11.912 -14.595 -17.507 -20.628 -23.887 -27.357 -31.033 -35.073 -39.589] % Datasheet derived  CapacityChangeThermal=[0, 0; 0, 0; 0, 0; 0, 0] % Parameter not set  CapacityChangeThermalI=repmat(0, 4, 2, 3) % Parameter not set  CapacityCyclingChangeInitialTarget=0 % Parameter not set  SelfDischargeRChangeVec=[0, 0, 0, 0] % Parameter not set  SelfDischargeRChangeThermal=[0, 0; 0, 0; 0, 0; 0, 0] % Parameter not set  SelfDischargeRChangeThermalI=repmat(0, 4, 2, 3) % Parameter not set  SelfDischargeRCyclingChangeInitialTarget=0 % Parameter not set  R1ChangeVec=[0, 0, 0, 0] % Parameter not set  R1ChangeThermal=[0, 0; 0, 0; 0, 0; 0, 0] % Parameter not set  R1ChangeThermalI=repmat(0, 4, 2, 3) % Parameter not set  R1CyclingChangeInitialTarget=0 % Parameter not set  R2ChangeVec=[0, 0, 0, 0] % Parameter not set  R2ChangeThermal=[0, 0; 0, 0; 0, 0; 0, 0] % Parameter not set  R2ChangeThermalI=repmat(0, 4, 2, 3) % Parameter not set  R2CyclingChangeInitialTarget=0 % Parameter not set  R3ChangeVec=[0, 0, 0, 0] % Parameter not set  R3ChangeThermal=[0, 0; 0, 0; 0, 0; 0, 0] % Parameter not set  R3ChangeThermalI=repmat(0, 4, 2, 3) % Parameter not set  R3CyclingChangeInitialTarget=0 % Parameter not set  CalendarAgeResistance=simscape.battery.enum.cells.BatteryEnable.Disabled  CalendarAgeCapacity=simscape.battery.enum.cells.BatteryEnable.Enabled  CalendarAgingMethod=simscape.battery.enum.cells.CalendarAgingMethod.tableTandTime  StorageVariable=simscape.battery.enum.cells.StorageVariable.OCV  OCVDuringStorage=0.9 % Parameter not set  SOCDuringStorage=0.6 % Parameter not set  StorageTimeIntervals=0 % Parameter not set d  StorageTemperatures=273 % Parameter not set K  ResistanceScalingOCV=2.2134e6 % Parameter not set  ResistanceScalingOCVOffset=1.632e6 % Parameter not set  ResistanceExponentialIncrease=0.515833569 % Parameter not set V  ResistanceTimeExponent=0.75 % Parameter not set  ResistanceAgeTemperatureBreakpoints=[273.15, 298.15, 323.15] % Parameter not set K  ResistanceAgeTimeBreakpoints=[0, 90, 180, 270] % Parameter not set d  PercentResistanceChange=[0, 0, 0] % Parameter not set  ResistanceTimeBreakpoints=100 % Parameter not set d  PercentResistanceChangeThermal=[0, 0, 0; 0, 0, 0; 0, 0, 0; 0, 0, 0] % Parameter not set  CapacityScalingOCV=1.5097e07 % Parameter not set  CapacityScalingOCVOffset=8.3625e06 % Parameter not set  CapacityExponentialIncrease=0.6011 % Parameter not set V  CapacityTimeExponent=0.75 % Parameter not set  CapacityAgeTemperatureBreakpoints=[5 25 30 40] % Datasheet derived degC  CapacityAgeTimeBreakpoints=[1 29 57 85 113 141 169 197 225 253 281 309 337 365 393 421 449 477 505 533 561] % Datasheet derived d  PercentCapacityChange=[0, 0, 0] % Parameter not set  CapacityTimeBreakpoints=100 % Parameter not set d  PercentCapacityChangeThermal=[-12.16003 -12.05239 -12.1695 -12.09683;-12.86337 -14.52728 -16.99685 -20.72464;-13.70598 -17.13684 -21.40096 -27.85651;-14.55234 -19.69649 -25.62782 -33.8946;-15.39921 -22.17854 -29.53628 -39.21373;-16.25192 -24.59585 -33.26735 -43.824;-17.06738 -27.04531 -36.69448 -48.04282;-17.84583 -29.39901 -39.91743 -51.10766;-18.67228 -31.83985 -42.90723 -53.76751;-19.4824 -34.22411 -45.64728 -56.42735;-20.29628 -36.48052 -48.11969 -59.0872;-21.15972 -38.79001 -50.6323 -61.74704;-21.98269 -40.98584 -53.11668 -64.40688;-22.7952 -43.14859 -55.60106 -67.06673;-23.58639 -45.35431 -58.08544 -69.72657;-24.41788 -47.50229 -60.56983 -72.38642;-25.26019 -49.69778 -63.05421 -75.04626;-26.10099 -51.98571 -65.53859 -77.7061;-26.91077 -54.29114 -68.02297 -80.36595;-27.73583 -56.59657 -70.50735 -83.02579;-28.55906 -58.902 -72.99173 -85.68564]  SimulationTemperature=298.15 % Parameter not set K  BatteryThermalMass=2340 % Parameter assumed J/K  NumThermalModels=6 % Parameter not set  ThermalConductivityZ=18 % Parameter not set W/(K*m)  CrossSectionalAreaXY=9784.8 % Datasheet derived mm^2  Height=94.3 % Datasheet derived mm  ReversibleHeatModel=simscape.battery.enum.cells.ReversibleHeatModel.Disabled  EntropicCoefficient=[0, 0, 0, 0, 0, 0, 0] % Parameter not set mV/K  CurrentDirectionality=simscape.battery.enum.cells.BatteryEnable.Disabled  stateOfCharge_specify=off  stateOfCharge_priority=High  stateOfCharge=1  stateOfCharge_nominal_specify=off  stateOfCharge_nominal_value=1  stateOfCharge_nominal_unit=1  batteryVoltage_specify=off  batteryVoltage_priority=None  batteryVoltage=0 V  batteryVoltage_nominal_specify=off  batteryVoltage_nominal_value=1  batteryVoltage_nominal_unit=V  batteryCurrent_specify=off  batteryCurrent_priority=None  batteryCurrent=0 A  batteryCurrent_nominal_specify=off  batteryCurrent_nominal_value=1  batteryCurrent_nominal_unit=A  numCycles_specify=off  numCycles_priority=High  numCycles=0  numCycles_nominal_specify=off  numCycles_nominal_value=1  numCycles_nominal_unit=1  batteryTemperature_specify=off  batteryTemperature_priority=High  batteryTemperature=298.15 K  batteryTemperature_nominal_specify=off  batteryTemperature_nominal_value=1  batteryTemperature_nominal_unit=K  hysteresisState_specify=off  hysteresisState_priority=High  hysteresisState=0  hysteresisState_nominal_specify=off  hysteresisState_nominal_value=1  hysteresisState_nominal_unit=1  isExothermFaulted_specify=off  isExothermFaulted_priority=None  isExothermFaulted=0  isExothermFaulted_nominal_specify=off  isExothermFaulted_nominal_value=1  isExothermFaulted_nominal_unit=1  reactionHeatRate_specify=off  reactionHeatRate_priority=None  reactionHeatRate=0 W  reactionHeatRate_nominal_specify=off  reactionHeatRate_nominal_value=1  reactionHeatRate_nominal_unit=W  reactionExtent_specify=off  reactionExtent_priority=None  reactionExtent=0  reactionExtent_nominal_specify=off  reactionExtent_nominal_value=1  reactionExtent_nominal_unit=1
      settings: AttributesFormatString=CSB Battery:GPL1272
  Buck Converter : ee_lib/Semiconductors & Converters/Converters/Buck Converter  port_option=ee.enum.controlport.ps  device_type=ee.enum.converters.switchingdevice.ideal  Vf=0.8 V  Ron=0.001 Ohm  Rds=0.001 Ohm  Goff=1e-5 1/Ohm  Vgt=1 V  Vgt_off=-1 V  Ih=1 A  Vth=6 V  K=0  diode_param=ee.enum.converters.protectiondiode.nodynamics  diode_Vf=0.8 V  diode_Ron=0.001 Ohm  diode_Goff=1e-5 1/Ohm  diode_C=50 nF  diode_iRM=-235 A  diode_iF=300 A  diode_idot=-50 A/us  diode_trr_param=ee.enum.converters.diodetrr.trr_factor  diode_trr_factor=3  diode_trr=15 us  diode_Qrr=1500 s*uA  Lf=1e-6 H  Rl=0 Ohm  Cf=1e-7 F  Rf=1e-6 Ohm  snubber_type=ee.enum.converters.snubber.exclude  Cs=1e-7 F  Rs=0.1 Ohm  iL_specify=off  iL_priority=High  iL=0 A  iL_nominal_specify=off  iL_nominal_value=1  iL_nominal_unit=A  vc_specify=off  vc_priority=High  vc=0 V  vc_nominal_specify=off  vc_nominal_value=1  vc_nominal_unit=V
  Bus Creator : BusCreator  Inputs=2
  Capacitor : fl_lib/Electrical/Electrical Elements/Capacitor  c=0.1 uF  r=0 Ohm  g=0 1/Ohm  i_specify=off  i_priority=None  i=0 A  i_nominal_specify=off  i_nominal_value=1  i_nominal_unit=A  v_specify=off  v_priority=None  v=0 V  v_nominal_specify=off  v_nominal_value=1  v_nominal_unit=V  vc_specify=off  vc_priority=High  vc=0 V  vc_nominal_specify=off  vc_nominal_value=1  vc_nominal_unit=V
      settings: AttributesFormatString=%<c>%<c_unit>
  Charge Controller : Subsystem
  Connection Label : ConnectionLabel  Label=SolarPos
  Current Sensor1 : fl_lib/Electrical/Electrical Sensors/Current Sensor
  DC Motor : ee_lib/Electromechanical/Brushed Motors/DC Motor  field_option=ee.enum.field_option.pm  Rf=100 Ohm  Lf=1 H  Laf=0.15 H  If0=0 A  parameterization=ee.enum.dcparam_option.circuit_param  Ra=3.9 Ohm  La=12e-6 H  emf_or_torque=ee.enum.emf_or_torque.kv  Kv=0.072e-3 V/rpm  Ki=6.876e-4 N*m/A  T_stall=0.24e-3 N*m  w_max=19100 rpm  w_rated=15000 rpm  P_rated=0.08 W  V_rated=1.5 V  lam_param=ee.enum.lam_param.damping  i_noload=0 A  V_i_noload=1.5 V  J=0.01 cm^2*g  lam=0 N*m*s/rad  speed0=0 rpm  alpha=3.93e-3 1/K  Tmeas=25 degC  thermal_mass=100 J/K  initial_temperature=25 degC
  DIY Synchronous Buck Converter : Subsystem
  Electrical Reference : fl_lib/Electrical/Electrical Elements/Electrical Reference
  Electrical Reference1 : fl_lib/Electrical/Electrical Elements/Electrical Reference
  Electrical Reference2 : fl_lib/Electrical/Electrical Elements/Electrical Reference
  Motor Controller : Subsystem
  PS-Simulink Converter : nesl_utility/PS-Simulink Converter  PhysicalDomain=network_engine_domain  SubClassName=ps_output  LeftPortType=input  RightPortType=output  PseudoPeriodic=off  Frequencies=[]  VectorFormat=inherit  Unit=inherit  AffineConversion=off
  PS-Simulink Converter1 : nesl_utility/PS-Simulink Converter  PhysicalDomain=network_engine_domain  SubClassName=ps_output  LeftPortType=input  RightPortType=output  PseudoPeriodic=off  Frequencies=[]  VectorFormat=inherit  Unit=inherit  AffineConversion=off
  PS-Simulink Converter2 : nesl_utility/PS-Simulink Converter  PhysicalDomain=network_engine_domain  SubClassName=ps_output  LeftPortType=input  RightPortType=output  PseudoPeriodic=off  Frequencies=[]  VectorFormat=inherit  Unit=inherit  AffineConversion=off
  Resistor : fl_lib/Electrical/Electrical Elements/Resistor  R=12 kOhm  i_specify=off  i_priority=None  i=0 A  i_nominal_specify=off  i_nominal_value=1  i_nominal_unit=A  v_specify=off  v_priority=None  v=0 V  v_nominal_specify=off  v_nominal_value=1  v_nominal_unit=V
      settings: AttributesFormatString=%<R> %<R_unit>
  Resistor1 : fl_lib/Electrical/Electrical Elements/Resistor  R=3 kOhm  i_specify=off  i_priority=None  i=0 A  i_nominal_specify=off  i_nominal_value=1  i_nominal_unit=A  v_specify=off  v_priority=None  v=0 V  v_nominal_specify=off  v_nominal_value=1  v_nominal_unit=V
      settings: AttributesFormatString=%<R> %<R_unit>
  Simulink-PS Converter : nesl_utility/Simulink-PS Converter  PhysicalDomain=network_engine_domain  SubClassName=ps_input  LeftPortType=input  RightPortType=output  PseudoPeriodic=off  Frequencies=[]  NoiseDistribution=none  NoiseParameters=[]  Unit=1  AffineConversion=off  FilteringAndDerivatives=provide  SimscapeFilterOrder=1  InputFilterTimeConstant=0.001  UdotUserProvided=0
  Solar Panel : ee_lib/Sources/Solar Cell  prm=ee.enum.sources.solar_cell_prm.datasheet  Isc=3.1 A  Voc=21.8 V  Is=1e-6 A  Is2=0 A  Iph=7.34 A  Ir0=1000 W/m^2  ec=1.5  N2=2  Rs=0 Ohm  Rp=inf Ohm  N_series=36  N_parallel=1  TIPH1=0 1/K  EG=1.11 eV  TXIS1=3  TXIS2=3  TRS1=0  TRP1=0  Tmeas=25 degC  TFIXED=25 degC  thermal_mass=100 J/K  initial_temperature=25 degC
  Solver Configuration : nesl_utility/Solver Configuration  PhysicalDomain=network_engine_domain  SubClassName=solver  LeftPortType=input  RightPortType=generic  Tones=[]  Harmonics=[]  SimulateNoise=off  Profile=off  UseLocalSampling=off  EnableSwitchedLinearOptims=on  FrequencyDomain=off  UseCCode=off  RelTol=0.001  AbsTol=0.001  MinStep=1e-09  ToWorkspace=off  RevertToSquareIcSolve=off  NumHomotopyIterations=100  PhasorMode=off  PhasorModeNumHarmonics=1  ConsistencySolver=NEWTON_XTOL_AFTER_FTOL  CanonicalOrdering=CANONICAL  OptimizeIntermediates=OPTIMIZED  IndexReductionMethod=DerivativeReplacement  DoDC=off  ResidualTolerance=1e-09  ConsistencyTolSource=GLOBAL  ConsistencyAbsTol=0.001  ConsistencyRelTol=0.001  ConsistencyTolFactor=0.001  UseLocalSolver=off  LocalSolverChoice=NE_BACKWARD_EULER_ADVANCER  ResolveIndetEquations=on  FunctionEvalNumThread=1  LocalSolverSampleTime=0.001  DoFixedCost=off  MaxNonlinIter=3  MaxModeIter=2  ComputeImpulses=off  ImpulseIterations=2  LinearAlgebra=auto  LinearAlgebraNumThread=0  EquationFormulation=NE_TIME_EF  DelaysMemoryBudget=1024  AutomaticFiltering=on  FilteringTimeConstant=0.001  PartitionStorageMethod=AS_NEEDED  PartitionMemoryBudget=1024  PartitionMethod=ROBUST  MultibodyUseLocalSolver=off  MultibodyLocalSolverChoice=ODE1  MultibodyLocalSolverSampleTime=0.001
  Voltage Sensor : fl_lib/Electrical/Electrical Sensors/Voltage Sensor
  Voltage Sensor1 : fl_lib/Electrical/Electrical Sensors/Voltage Sensor
  wires:
  PS-Simulink Converter/1 -> [PV_I]  "PV_I"
  PS-Simulink Converter1/1 -> [PV_V]  "PV_V"
  Charge Controller/1(Out1) -> Simulink-PS Converter/1  "PWM"
  [PV_V] -> Bus Creator/1
  [PV_I] -> Bus Creator/2
  Bus Creator/1 -> Charge Controller/1(In1)  "PV_Data_Bus"
  PS-Simulink Converter2/1 -> [Bat_V_Div]
  [Bat_V_Div] -> Charge Controller/2(Bat_V_Div)
  connections:
  Electrical Reference/LConn1 -- Buck Converter/LConn3 -- Voltage Sensor1/RConn2 -- Solar Panel/RConn1
  Current Sensor1/RConn2 -- Buck Converter/LConn2 -- Voltage Sensor1/LConn1 -- Connection Label/LConn1
  Current Sensor1/LConn1 -- Solar Panel/LConn2
  PS-Simulink Converter/LConn1 -- Current Sensor1/RConn1
  PS-Simulink Converter1/LConn1 -- Voltage Sensor1/RConn1
  Simulink-PS Converter/RConn1 -- Buck Converter/LConn1
  Electrical Reference1/LConn1 -- Resistor1/RConn1 -- Capacitor/RConn1 -- Buck Converter/RConn2 -- Battery Equivalent Circuit1/RConn1
  Buck Converter/RConn1 -- Resistor/LConn1 -- Battery Equivalent Circuit1/LConn1
  Resistor/RConn1 -- Voltage Sensor/LConn1 -- Capacitor/LConn1 -- Resistor1/LConn1
  Electrical Reference2/LConn1 -- Voltage Sensor/RConn2
  PS-Simulink Converter2/LConn1 -- Voltage Sensor/RConn1
